simulink model "open_loop"  (R2021b)
settings: Solver=VariableStepAuto  StartTime=0.0  StopTime=5  RelTol=1e-3
values from neighbouring files (symbols this model uses):
  A = [0, 0, 0, 1, 0, 0 ... (first row only)    [basic_data.m]    (also in basic_data.mat = [0 0 0 0 -22.4688936865 5 0 0 0 6.5 19.3959496459 -3.6 ... (; lqr.mat = [0 0 0 0 -22.4688936865 5 0 0 0 6.5 19.3959496459 -3.6 ... ()
  B = [0, 0 ... (first row only)    [basic_data.m]    (also in basic_data.mat = [0  0; 0  0; 0  0; 27  11.2; 6.06660129535  -1.63757677119; ; lqr.mat = [0  0; 0  0; 0  0; 27  11.2; 6.06660129535  -1.63757677119; )
  x_0 = [0.2, -0.1, 0.15, -1, 0.8, 0]'    [basic_data.m]    (also in basic_data.mat = [0.2 -0.1 0.15 -1 0.8 0]; lqr.mat = [0.2 -0.1 0.15 -1 0.8 0])
settings Model: Creator=asus  LastModifiedBy=asus

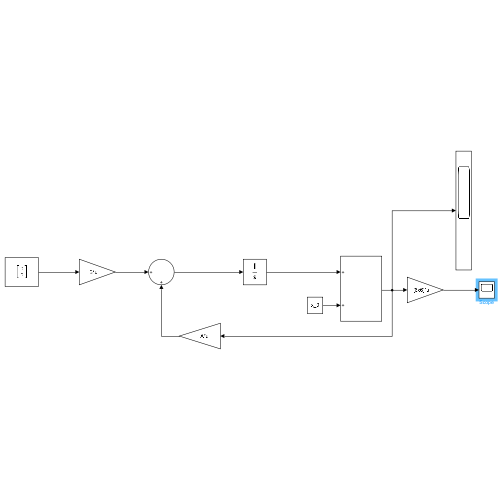
[thumbnail: Simulink's stored preview of the top-level diagram]
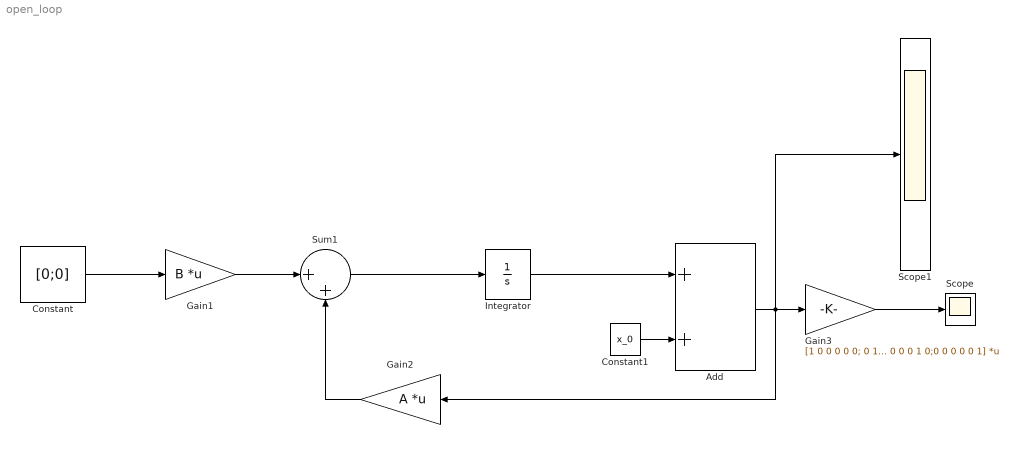
== system open_loop ==
  Add : Sum
  Constant : Constant  Value=[0;0]  VectorParams1D=off
  Constant1 : Constant  Value=x_0  VectorParams1D=off
  Gain1 : Gain  Gain=B  Multiplication=Matrix(K*u)
  Gain2 : Gain  Gain=A  Multiplication=Matrix(K*u)
  Gain3 : Gain  Gain=[1 0 0 0 0 0; 0 1 0 0 0 0;0 0 1 0 0 0;0 0 0 1 0 0;0 0 0 0 1 0;0 0 0 0 0 1]  Multiplication=Matrix(K*u)
  Integrator : Integrator
  Scope : Scope
  Scope1 : Scope
  Sum1 : Sum  Inputs=|++
  wires:
  Integrator/1 -> Add/1
  Sum1/1 -> Integrator/1
  Constant/1 -> Gain1/1
  Gain1/1 -> Sum1/1
  Gain2/1 -> Sum1/2
  Gain3/1 -> Scope/1
  Constant1/1 -> Add/2
  Add/1 -> Scope1/1, Gain2/1, Gain3/1
